simulink model "quadRotorController"  (R2023a)
settings: Solver=VariableStepAuto  StartTime=0.0  StopTime=100  RelTol=1e-3  EnableMultiTasking=on
libraries: simulink x1
settings Model: Creator=Nariman  LastModifiedBy=juanv
settings SolverCC: AlgebraicLoopSolver=TrustRegion
settings DataIOCC: ReturnWorkspaceOutputs=off
settings OptimizationCC: LifeSpan=inf
settings DebuggingCC: UnconnectedInputMsg=warning  UnconnectedOutputMsg=warning  UnconnectedLineMsg=warning  SFUnexpectedBacktrackingDiag=warning  SFNoUnconditionalDefaultTransitionDiag=warning  ArithmeticOperatorsInVariantConditions=warning
settings ModelReferenceCC: EnableRefExpFcnMdlSchedulingChecks=on
settings SFSimCC: SimUseLocalCustomCode=off  CustomCodeUndefinedFunction=UseInterfaceOnly
settings RTWCC: RTWUseLocalCustomCode=off
settings CodeAppCC: StateflowObjectComments=on
settings GRTTargetCC: TargetLangStandard=C89/C90 (ANSI)
settings ConfigComp: CovMetricSettings=dw  CovSaveCumulativeToWorkspaceVar=on  CovSaveSingleToWorkspaceVar=on  CovExternalEMLEnable=off

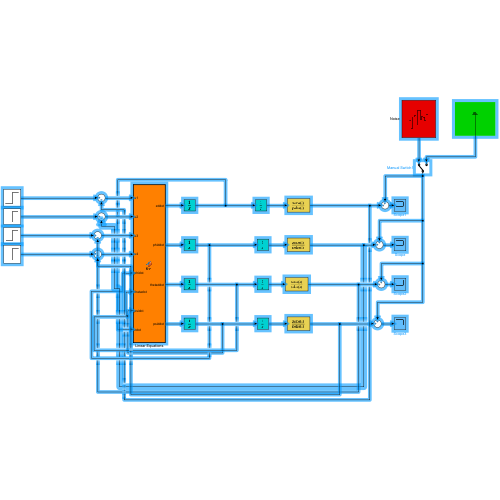
[thumbnail: Simulink's stored preview of the top-level diagram]
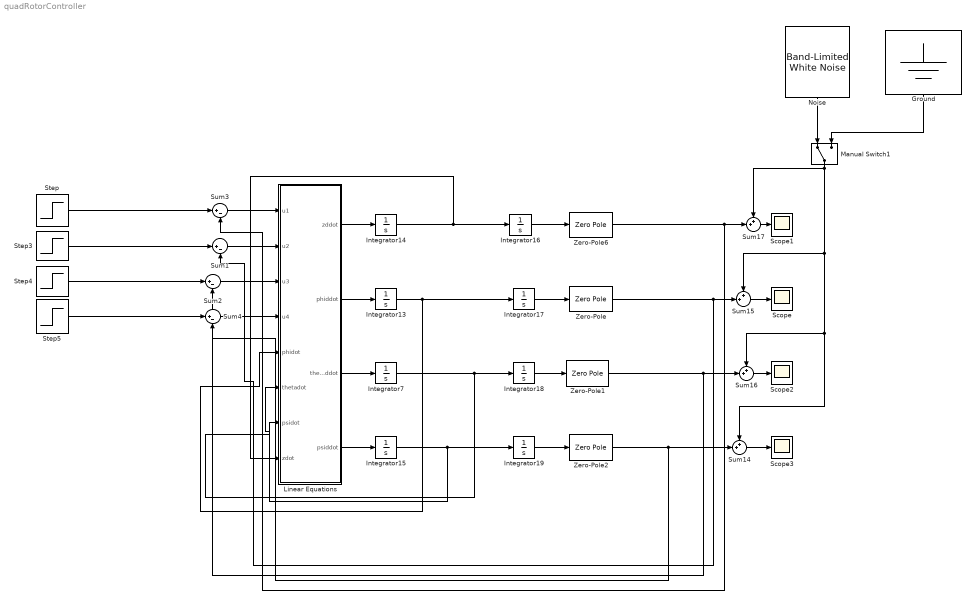
== system quadRotorController ==
  Ground : Ground
  Integrator{7,13..19} (8 alike) : Integrator
  Linear Equations : MATLAB Function  TreatAsAtomicUnit=on
  Manual Switch1 : ManualSwitch
  Noise : simulink/Sources/Band-Limited White Noise  Cov=0.0000000001  Ts=0.1  seed=[23341]
  Scope{,1..3} (4 alike) : Scope
  Step{,3..5} (4 alike) : Step  After=0.01  SampleTime=0
  Sum{1..4} (4 alike) : Sum  Inputs=|+-
  Sum{14..17} (4 alike) : Sum  Inputs=++|
  Zero-Pole : ZeroPole  Zeros=[-0.949]  Poles=[-49]  Gain=[290]
  Zero-Pole1 : ZeroPole  Zeros=[-0.949]  Poles=[-49]  Gain=[100]
  Zero-Pole2 : ZeroPole  Zeros=[-0.3]  Poles=[-16.1]  Gain=[3.58]
  Zero-Pole6 : ZeroPole  Zeros=[-0.3]  Poles=[-16.1]  Gain=[90.58]
  wires:
  Linear Equations/4(psiddot) -> Integrator15/1
  Linear Equations/3(thetaddot) -> Integrator7/1
  Linear Equations/2(phiddot) -> Integrator13/1
  Linear Equations/1(zddot) -> Integrator14/1
  Integrator15/1 -> Linear Equations/7(psidot), Integrator19/1
  Integrator7/1 -> Linear Equations/6(thetadot), Integrator18/1
  Integrator13/1 -> Integrator17/1, Linear Equations/5(phidot)
  Integrator14/1 -> Integrator16/1, Linear Equations/8(zdot)
  Integrator17/1 -> Zero-Pole/1
  Integrator18/1 -> Zero-Pole1/1
  Zero-Pole/1 -> Sum15/2, Sum1/2
  Sum3/1 -> Linear Equations/1(u1)
  Step/1 -> Sum3/1
  Sum1/1 -> Linear Equations/2(u2)
  Sum2/1 -> Linear Equations/3(u3)
  Sum4/1 -> Linear Equations/4(u4)
  Zero-Pole1/1 -> Sum16/2, Sum2/2
  Integrator19/1 -> Zero-Pole2/1
  Zero-Pole2/1 -> Sum14/2, Sum4/2
  Integrator16/1 -> Zero-Pole6/1
  Zero-Pole6/1 -> Sum17/2, Sum3/2
  Noise/1 -> Manual Switch1/1
  Ground/1 -> Manual Switch1/2
  Sum14/1 -> Scope3/1
  Sum17/1 -> Scope1/1
  Sum16/1 -> Scope2/1
  Sum15/1 -> Scope/1
  Manual Switch1/1 -> Sum17/1, Sum15/1, Sum16/1, Sum14/1
  Step3/1 -> Sum1/1
  Step4/1 -> Sum2/1
  Step5/1 -> Sum4/1

== matlab function quadRotorController/Linear Equations ==
  data: u1 input; zddot output; u2 input; u3 input; u4 input; phidot input; thetadot input; psidot input; phiddot output; thetaddot output; psiddot output; zdot input
function [zddot,phiddot,thetaddot,psiddot] = fcn(u1,u2,u3,u4,phidot,thetadot,psidot,zdot)
ixx=0.0086;
iyy=0.0086;
izz=0.0176;
m=0.47;
zddot=zdot+u1/m;
phiddot=phidot+u2/ixx;
thetaddot=thetadot+u3/iyy;
psiddot=psidot+u4/izz;
